simulink model "ASM1_Influentmodel1_ff_calibration"  (Simulink 8.0)
settings: Solver=ode45  StartTime=0.0  StopTime=146  RelTol=1e-5
undefined symbols (not defined in the file or in its folder): Ccj_gperPEperd, Ccj_HH_max, Ccj_HH_min, Ccj_HH_ns, Ccj_HH_nv, Ccj_HH_st, Cli_gperPEperd, Cli_HH_max, Cli_HH_min, Cli_HH_ns, Cli_HH_nv, Cli_HH_st, CODpart_gperPEperd, CODpart_HH_max, CODpart_HH_min, CODpart_HH_ns, CODpart_HH_nv, CODpart_HH_st, CODpart_Ind_kgperd, CODpart_Ind_max, CODpart_Ind_min, CODpart_Ind_ns, CODpart_Ind_nv, CODpart_Ind_st, CODsol_gperPEperd, CODsol_HH_max, CODsol_HH_min, CODsol_HH_ns, CODsol_HH_nv, CODsol_HH_st, CODsol_Ind_kgperd, CODsol_Ind_max, CODsol_Ind_min, CODsol_Ind_ns, CODsol_Ind_nv, CODsol_Ind_st, Csl_gperPEperd, Csl_HH_max, Csl_HH_min, Csl_HH_ns, Csl_HH_nv, Csl_HH_st, Csl_i_gperPEperd, Csl_i_HH_max, Csl_i_HH_min, Csl_i_HH_ns, Csl_i_HH_nv, Csl_i_HH_st, FFfraction, HHpolnoiseswitch, HHpopswitch, Indpolnoiseswitch, Indpopswitch, PE, polnoiseswitch, SI_max, SI_min, SI_ns, SI_nv, SI_st ... (+73)
Description:
  | BSM2 influent model, version 15 March 2005
settings Model: Creator=Krist V. Gernaey  LastModifiedBy=lasn  ExtModeAutoUpdateStatusClock=off
settings DataIOCC: LimitDataPoints=off  SignalLoggingSaveFormat=ModelDataLogs  SignalLoggingName=sigsOut  OutputOption=SpecifiedOutputTimes  OutputTimes=[0:1/96:146]
settings OptimizationCC: InitFltsAndDblsToZero=on
settings DebuggingCC: SaveWithParameterizedLinksMsg=none  SignalResolutionControl=TryResolveAllWithWarning  SolverPrmCheckMsg=none  MultiTaskDSMMsg=warning  MultiTaskCondExecSysMsg=none  FcnCallInpInsideContextMsg=UseLocalSettings  StrictBusMsg=None
settings HardwareCC: TargetEndianess=LittleEndian  TargetHWDeviceType=MATLAB Host  ProdEqTarget=off
settings RTWCC: IncludeERTFirstTime=on
settings GRTTargetCC: CombineOutputUpdateFcns=off  GRTInterface=on

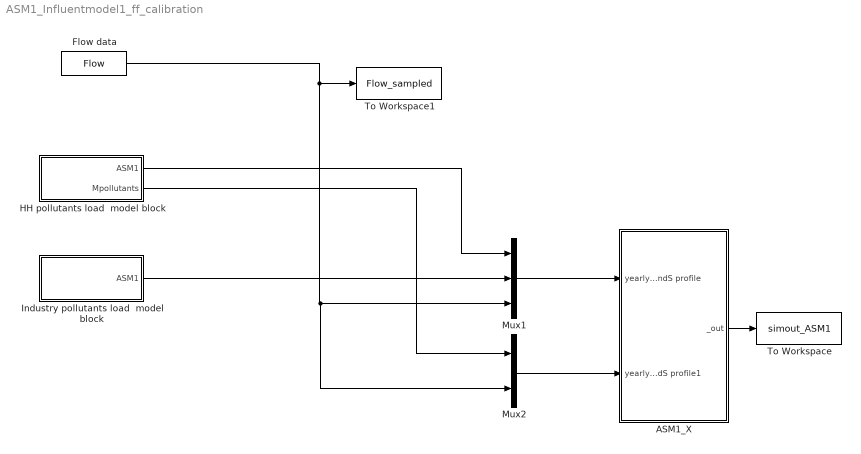
== system ASM1_Influentmodel1_ff_calibration ==
  ASM1_X : Subsystem
  Flow data : FromWorkspace  VariableName=Flow  SampleTime=(1/24)
  "HH pollutants load  model block " : Subsystem
  "Industry pollutants load  model block " : Subsystem
  Mux1 : Mux  Inputs=3
  Mux2 : Mux  Inputs=2
  To Workspace : ToWorkspace  VariableName=simout_ASM1  SampleTime=-1
  To Workspace1 : ToWorkspace  VariableName=Flow_sampled  SampleTime=-1
  wires:
  "HH pollutants load  model block "/1(ASM1) -> Mux1/1
  Mux1/1 -> ASM1_X/1(yearly_indS profile)
  ASM1_X/1(_out) -> To Workspace/1
  "HH pollutants load  model block "/2(Mpollutants) -> Mux2/1
  Mux2/1 -> ASM1_X/2(yearly_indS profile1)
  Flow data/1 -> To Workspace1/1, Mux2/2, Mux1/3
  "Industry pollutants load  model block "/1(ASM1) -> Mux1/2

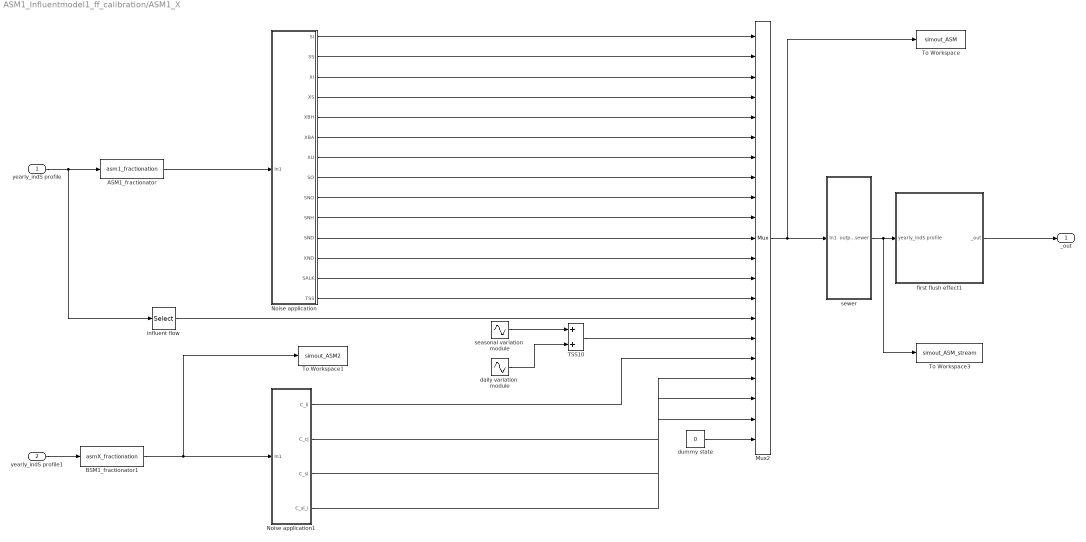
== system ASM1_Influentmodel1_ff_calibration/ASM1_X ==
  yearly_indS profile : Inport
  yearly_indS profile1 : Inport  Port=2
  ASM1_fractionator : S-Function  FunctionName=asm1_fractionation  Parameters=ASM1_PARS, ASM1_FRACTIONS  EnableBusSupport=off
  BSM1_fractionator1 : S-Function  FunctionName=asmX_fractionation  EnableBusSupport=off
  Mux2 : Mux  Inputs=21
  Noise application : Subsystem
  Noise application1 : Subsystem
  TSS10 : Sum
  To Workspace : ToWorkspace  VariableName=simout_ASM  SampleTime=-1
  To Workspace1 : ToWorkspace  VariableName=simout_ASM2  SampleTime=-1
  To Workspace3 : ToWorkspace  VariableName=simout_ASM_stream  SampleTime=-1
  daily variation  module : Sin  Amplitude=TdAmp  Bias=TdBias  Frequency=TdFreq  Phase=TdPhase  SampleTime=0
  "dummy state " : Constant  Value=0
  first flush effect1 : Subsystem
  influent flow : Selector  InputPortWidth=11  IndexOptions=Index vector (dialog)  Indices=[11]  OutputSizes=1
  seasonal variation  module : Sin  Amplitude=TAmp  Bias=TBias  Frequency=TFreq  Phase=TPhase  SampleTime=0
  sewer : Subsystem
  _out : Outport
  wires:
  yearly_indS profile/1 -> influent flow/1, ASM1_fractionator/1
  ASM1_fractionator/1 -> Noise application/1(In1)
  Mux2/1 -> sewer/1(In1), To Workspace/1
  Noise application1/1(C_li) -> Mux2/17
  Noise application/2(SS) -> Mux2/2
  Noise application/1(SI) -> Mux2/1
  Noise application/8(SO) -> Mux2/8
  Noise application/9(SNO) -> Mux2/9
  Noise application/10(SNH) -> Mux2/10
  Noise application/11(SND) -> Mux2/11
  Noise application/12(XND) -> Mux2/12
  seasonal variation  module/1 -> TSS10/1
  daily variation  module/1 -> TSS10/2
  TSS10/1 -> Mux2/16
  yearly_indS profile1/1 -> BSM1_fractionator1/1
  BSM1_fractionator1/1 -> Noise application1/1(In1), To Workspace1/1
  Noise application1/2(C_cj) -> Mux2/18
  Noise application1/3(C_sl) -> Mux2/19
  Noise application1/4(C_sl_i) -> Mux2/20
  "dummy state "/1 -> Mux2/21
  Noise application/3(XI) -> Mux2/3
  Noise application/4(XS) -> Mux2/4
  Noise application/5(XBH) -> Mux2/5
  Noise application/6(XBA) -> Mux2/6
  Noise application/7(XU) -> Mux2/7
  Noise application/13(SALK) -> Mux2/13
  Noise application/14(TSS) -> Mux2/14
  influent flow/1 -> Mux2/15
  sewer/1(output sewer) -> To Workspace3/1, first flush effect1/1(yearly_indS profile)
  first flush effect1/1(_out) -> _out/1

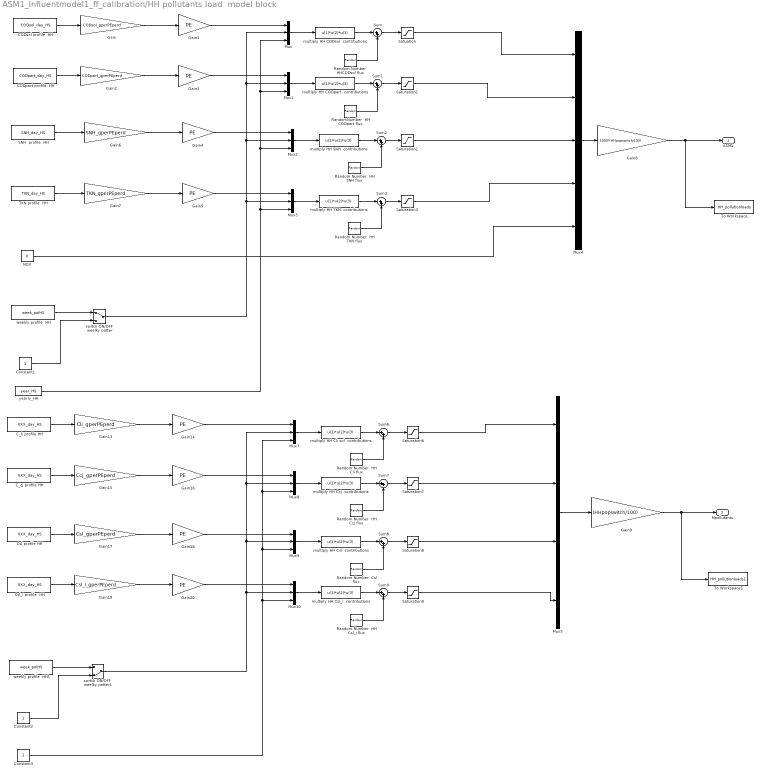
== system ASM1_Influentmodel1_ff_calibration/HH pollutants load  model block  ==
  CODpart profile  HH : FromWorkspace  VariableName=CODpart_day_HS  SampleTime=1/24  Interpolate=off  OutputAfterFinalValue=Cyclic repetition
  CODsol profile  HH : FromWorkspace  VariableName=CODsol_day_HS  SampleTime=1/24  Interpolate=off  OutputAfterFinalValue=Cyclic repetition
  C_cj profile HH : FromWorkspace  VariableName=XXX_day_HS  SampleTime=1/24  Interpolate=off  OutputAfterFinalValue=Cyclic repetition
  C_li profile HH : FromWorkspace  VariableName=XXX_day_HS  SampleTime=1/24  Interpolate=off  OutputAfterFinalValue=Cyclic repetition
  Constant1 : Constant
  Constant2 : Constant
  Constant3 : Constant
  Csl profile HH : FromWorkspace  VariableName=XXX_day_HS  SampleTime=1/24  Interpolate=off  OutputAfterFinalValue=Cyclic repetition
  Csl_I profile  HH : FromWorkspace  VariableName=XXX_day_HS  SampleTime=1/24  Interpolate=off  OutputAfterFinalValue=Cyclic repetition
  Gain : Gain  Gain=CODsol_gperPEperd
  Gain{1,3..5,14,16,18,20} (8 alike) : Gain  Gain=PE
  Gain13 : Gain  Gain=Cli_gperPEperd
  Gain15 : Gain  Gain=Ccj_gperPEperd
  Gain17 : Gain  Gain=Csl_gperPEperd
  Gain19 : Gain  Gain=Csl_i_gperPEperd
  Gain2 : Gain  Gain=CODpart_gperPEperd
  Gain6 : Gain  Gain=SNH_gperPEperd
  Gain7 : Gain  Gain=TKN_gperPEperd
  Gain8 : Gain  Gain=1000*(HHpopswitch/100)
  Gain9 : Gain  Gain=(HHpopswitch/100)
  Mux{,1..3,7..10} (8 alike) : Mux  Inputs=3
  Mux4 : Mux  Inputs=5
  Mux5 : Mux
  NOX : Constant  Value=0
  Random Number  Csl flux : RandomNumber  Variance=Csl_HH_nv*HHpolnoiseswitch  Seed=Csl_HH_ns  SampleTime=Csl_HH_st
  Random Number  HH Ccj flux : RandomNumber  Variance=Ccj_HH_nv*HHpolnoiseswitch  Seed=Ccj_HH_ns  SampleTime=Ccj_HH_st
  Random Number  HH Cli flux : RandomNumber  Variance=Cli_HH_nv*HHpolnoiseswitch  Seed=Cli_HH_ns  SampleTime=Cli_HH_st
  Random Number  HH Csl_i flux : RandomNumber  Variance=Csl_i_HH_nv*HHpolnoiseswitch  Seed=Csl_i_HH_ns  SampleTime=Csl_i_HH_st
  Random Number  HH SNH flux : RandomNumber  Variance=SNH_HH_nv*HHpolnoiseswitch  Seed=SNH_HH_ns  SampleTime=SNH_HH_st
  Random Number  HH TKN flux : RandomNumber  Variance=TKN_HH_nv*HHpolnoiseswitch  Seed=TKN_HH_ns  SampleTime=TKN_HH_st
  Random Number  HHCODsol flux : RandomNumber  Variance=CODsol_HH_nv*HHpolnoiseswitch  Seed=CODsol_HH_ns  SampleTime=CODsol_HH_st
  RandomNumber  HH CODpart flux : RandomNumber  Variance=CODpart_HH_nv*HHpolnoiseswitch  Seed=CODpart_HH_ns  SampleTime=CODpart_HH_st
  SNH  profile  HH : FromWorkspace  VariableName=SNH_day_HS  SampleTime=1/24  Interpolate=off  OutputAfterFinalValue=Cyclic repetition
  Satuation : Saturate  UpperLimit=CODsol_HH_max  LowerLimit=CODsol_HH_min
  Saturation1 : Saturate  UpperLimit=CODpart_HH_max  LowerLimit=CODpart_HH_min
  Saturation2 : Saturate  UpperLimit=SNH_HH_max  LowerLimit=SNH_HH_min
  Saturation3 : Saturate  UpperLimit=TKN_HH_max  LowerLimit=TKN_HH_min
  Saturation6 : Saturate  UpperLimit=Cli_HH_max  LowerLimit=Cli_HH_min
  Saturation7 : Saturate  UpperLimit=Ccj_HH_max  LowerLimit=Ccj_HH_min
  Saturation8 : Saturate  UpperLimit=Csl_HH_max  LowerLimit=Csl_HH_min
  Saturation9 : Saturate  UpperLimit=Csl_i_HH_max  LowerLimit=Csl_i_HH_min
  Sum{,1..3,6..9} (8 alike) : Sum  Inputs=|++
  TKN profile  HH : FromWorkspace  VariableName=TKN_day_HS  SampleTime=1/24  Interpolate=off  OutputAfterFinalValue=Cyclic repetition
  To Workspace : ToWorkspace  VariableName=HH_pollutionloads  SampleTime=-1
  To Workspace1 : ToWorkspace  VariableName=HH_pollutionloads1  SampleTime=-1
  multiply HH CODpart  contributions : Fcn  Expr=u(1)*u(2)*u(3)
  multiply HH CODsol  contributions : Fcn  Expr=u(1)*u(2)*u(3)
  multiply HH Ccj  contributions : Fcn  Expr=u(1)*u(2)*u(3)
  multiply HH Cli sol  contributions : Fcn  Expr=u(1)*u(2)*u(3)
  multiply HH Csl  contributions : Fcn  Expr=u(1)*u(2)*u(3)
  multiply HH Csl_i  contributions : Fcn  Expr=u(1)*u(2)*u(3)
  multiply HH SNH  contributions : Fcn  Expr=u(1)*u(2)*u(3)
  multiply HH TKN  contributions : Fcn  Expr=u(1)*u(2)*u(3)
  switch ON/OFF  weelky patter : ManualSwitch
  switch ON/OFF  weelky patter1 : ManualSwitch  CurrentSetting=0
  weekly profile  HH : FromWorkspace  VariableName=week_polHS  SampleTime=1  Interpolate=off  OutputAfterFinalValue=Cyclic repetition
  weekly profile  HH1 : FromWorkspace  VariableName=week_polHS  SampleTime=1  Interpolate=off  OutputAfterFinalValue=Cyclic repetition
  yearly_HH : FromWorkspace  VariableName=year_HS  SampleTime=1  Interpolate=off  OutputAfterFinalValue=Cyclic repetition
  ASM1 : Outport
  Mpollutants : Outport  Port=2
  wires:
  Random Number  HHCODsol flux/1 -> Sum/2
  CODsol profile  HH/1 -> Gain/1
  Gain/1 -> Gain1/1
  Mux/1 -> multiply HH CODsol  contributions/1
  multiply HH CODsol  contributions/1 -> Sum/1
  Sum/1 -> Satuation/1
  Gain1/1 -> Mux/1
  RandomNumber  HH CODpart flux/1 -> Sum1/2
  CODpart profile  HH/1 -> Gain2/1
  Gain2/1 -> Gain3/1
  Mux1/1 -> multiply HH CODpart  contributions/1
  multiply HH CODpart  contributions/1 -> Sum1/1
  Sum1/1 -> Saturation1/1
  Gain3/1 -> Mux1/1
  Random Number  HH SNH flux/1 -> Sum2/2
  SNH  profile  HH/1 -> Gain6/1
  Gain6/1 -> Gain4/1
  Mux2/1 -> multiply HH SNH  contributions/1
  multiply HH SNH  contributions/1 -> Sum2/1
  Sum2/1 -> Saturation2/1
  Gain4/1 -> Mux2/1
  Random Number  HH TKN flux/1 -> Sum3/2
  TKN profile  HH/1 -> Gain7/1
  Gain7/1 -> Gain5/1
  Mux3/1 -> multiply HH TKN  contributions/1
  multiply HH TKN  contributions/1 -> Sum3/1
  Sum3/1 -> Saturation3/1
  Gain5/1 -> Mux3/1
  Mux4/1 -> Gain8/1
  Constant1/1 -> switch ON/OFF  weelky patter/2
  weekly profile  HH/1 -> switch ON/OFF  weelky patter/1
  Satuation/1 -> Mux4/1
  Saturation1/1 -> Mux4/2
  Saturation2/1 -> Mux4/3
  Saturation3/1 -> Mux4/4
  NOX/1 -> Mux4/5
  switch ON/OFF  weelky patter/1 -> Mux2/2, Mux/2, Mux1/2, Mux3/2
  yearly_HH/1 -> Mux2/3, Mux/3, Mux1/3, Mux3/3
  Gain8/1 -> ASM1/1, To Workspace/1
  Random Number  HH Cli flux/1 -> Sum6/2
  C_li profile HH/1 -> Gain13/1
  Gain13/1 -> Gain14/1
  Mux7/1 -> multiply HH Cli sol  contributions/1
  multiply HH Cli sol  contributions/1 -> Sum6/1
  Sum6/1 -> Saturation6/1
  Gain14/1 -> Mux7/1
  Random Number  HH Ccj flux/1 -> Sum7/2
  C_cj profile HH/1 -> Gain15/1
  Gain15/1 -> Gain16/1
  Mux8/1 -> multiply HH Ccj  contributions/1
  multiply HH Ccj  contributions/1 -> Sum7/1
  Sum7/1 -> Saturation7/1
  Gain16/1 -> Mux8/1
  Constant2/1 -> switch ON/OFF  weelky patter1/2
  weekly profile  HH1/1 -> switch ON/OFF  weelky patter1/1
  Random Number  Csl flux/1 -> Sum8/2
  Csl profile HH/1 -> Gain17/1
  Gain17/1 -> Gain18/1
  Mux9/1 -> multiply HH Csl  contributions/1
  multiply HH Csl  contributions/1 -> Sum8/1
  Sum8/1 -> Saturation8/1
  Gain18/1 -> Mux9/1
  Random Number  HH Csl_i flux/1 -> Sum9/2
  Csl_I profile  HH/1 -> Gain19/1
  Gain19/1 -> Gain20/1
  Mux10/1 -> multiply HH Csl_i  contributions/1
  multiply HH Csl_i  contributions/1 -> Sum9/1
  Sum9/1 -> Saturation9/1
  Gain20/1 -> Mux10/1
  switch ON/OFF  weelky patter1/1 -> Mux7/2, Mux8/2, Mux9/2, Mux10/2
  Saturation9/1 -> Mux5/4
  Saturation8/1 -> Mux5/3
  Saturation7/1 -> Mux5/2
  Saturation6/1 -> Mux5/1
  Mux5/1 -> Gain9/1
  Gain9/1 -> Mpollutants/1, To Workspace1/1
  Constant3/1 -> Mux7/3, Mux8/3, Mux9/3, Mux10/3

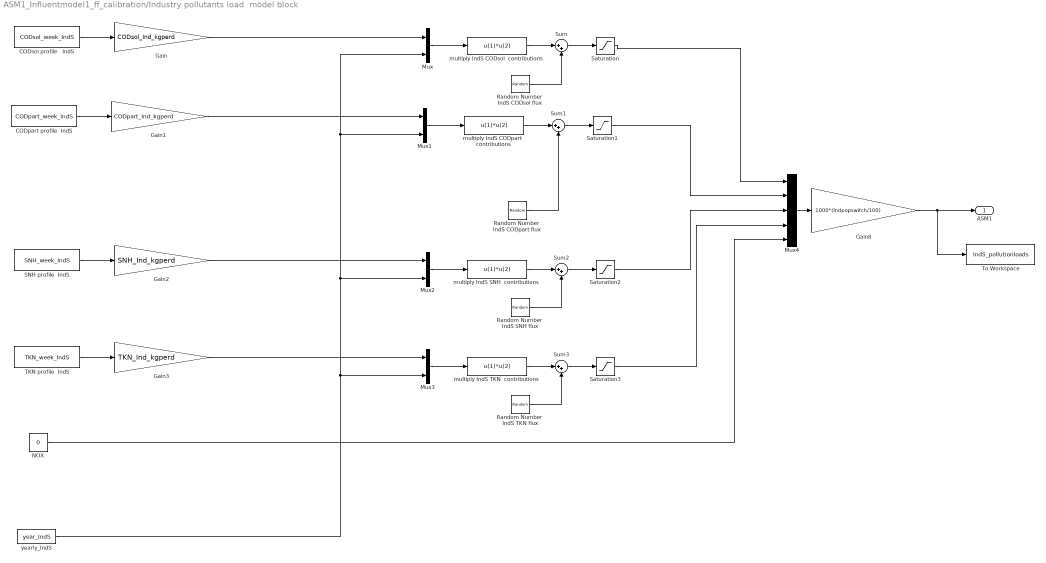
== system ASM1_Influentmodel1_ff_calibration/Industry pollutants load  model block  ==
  CODpart profile  IndS : FromWorkspace  VariableName=CODpart_week_IndS  SampleTime=1/6  Interpolate=off  OutputAfterFinalValue=Cyclic repetition
  CODsol profile   IndS : FromWorkspace  VariableName=CODsol_week_IndS  SampleTime=1/6  Interpolate=off  OutputAfterFinalValue=Cyclic repetition
  Gain : Gain  Gain=CODsol_Ind_kgperd
  Gain1 : Gain  Gain=CODpart_Ind_kgperd
  Gain2 : Gain  Gain=SNH_Ind_kgperd
  Gain3 : Gain  Gain=TKN_Ind_kgperd
  Gain8 : Gain  Gain=1000*(Indpopswitch/100)
  Mux{,1..3} (4 alike) : Mux  Inputs=2
  Mux4 : Mux  Inputs=5
  NOX : Constant  Value=0
  Random Number  IndS CODpart flux : RandomNumber  Variance=CODpart_Ind_nv*Indpolnoiseswitch  Seed=CODpart_Ind_ns  SampleTime=CODpart_Ind_st
  Random Number  IndS CODsol flux : RandomNumber  Variance=CODsol_Ind_nv*Indpolnoiseswitch  Seed=CODsol_Ind_ns  SampleTime=CODsol_Ind_st
  Random Number  IndS SNH flux : RandomNumber  Variance=SNH_Ind_nv*Indpolnoiseswitch  Seed=SNH_Ind_ns  SampleTime=SNH_Ind_st
  Random Number  IndS TKN flux : RandomNumber  Variance=TKN_Ind_nv*Indpolnoiseswitch  Seed=TKN_Ind_ns  SampleTime=TKN_Ind_st
  SNH profile  IndS : FromWorkspace  VariableName=SNH_week_IndS  SampleTime=1/6  Interpolate=off  OutputAfterFinalValue=Cyclic repetition
  Saturation : Saturate  UpperLimit=CODsol_Ind_max  LowerLimit=CODsol_Ind_min
  Saturation1 : Saturate  UpperLimit=CODpart_Ind_max  LowerLimit=CODpart_Ind_min
  Saturation2 : Saturate  UpperLimit=SNH_Ind_max  LowerLimit=SNH_Ind_min
  Saturation3 : Saturate  UpperLimit=TKN_Ind_max  LowerLimit=TKN_Ind_min
  Sum{,1..3} (4 alike) : Sum  Inputs=|++
  TKN profile  IndS : FromWorkspace  VariableName=TKN_week_IndS  SampleTime=1/6  Interpolate=off  OutputAfterFinalValue=Cyclic repetition
  To Workspace : ToWorkspace  VariableName=IndS_pollutionloads  SampleTime=-1
  multiply IndS CODpart  contributions : Fcn  Expr=u(1)*u(2)
  multiply IndS CODsol  contributions : Fcn  Expr=u(1)*u(2)
  multiply IndS SNH  contributions : Fcn  Expr=u(1)*u(2)
  multiply IndS TKN  contributions : Fcn  Expr=u(1)*u(2)
  yearly_IndS : FromWorkspace  VariableName=year_IndS  SampleTime=1  Interpolate=off  OutputAfterFinalValue=Cyclic repetition
  ASM1 : Outport
  wires:
  Random Number  IndS CODsol flux/1 -> Sum/2
  CODsol profile   IndS/1 -> Gain/1
  Mux/1 -> multiply IndS CODsol  contributions/1
  multiply IndS CODsol  contributions/1 -> Sum/1
  Sum/1 -> Saturation/1
  Mux4/1 -> Gain8/1
  Gain/1 -> Mux/1
  Random Number  IndS CODpart flux/1 -> Sum1/2
  CODpart profile  IndS/1 -> Gain1/1
  Mux1/1 -> multiply IndS CODpart  contributions/1
  multiply IndS CODpart  contributions/1 -> Sum1/1
  Sum1/1 -> Saturation1/1
  Gain1/1 -> Mux1/1
  Random Number  IndS SNH flux/1 -> Sum2/2
  SNH profile  IndS/1 -> Gain2/1
  Mux2/1 -> multiply IndS SNH  contributions/1
  multiply IndS SNH  contributions/1 -> Sum2/1
  Sum2/1 -> Saturation2/1
  Gain2/1 -> Mux2/1
  Random Number  IndS TKN flux/1 -> Sum3/2
  TKN profile  IndS/1 -> Gain3/1
  Mux3/1 -> multiply IndS TKN  contributions/1
  multiply IndS TKN  contributions/1 -> Sum3/1
  Sum3/1 -> Saturation3/1
  Gain3/1 -> Mux3/1
  yearly_IndS/1 -> Mux3/2, Mux2/2, Mux/2, Mux1/2
  Saturation/1 -> Mux4/1
  Saturation1/1 -> Mux4/2
  Saturation2/1 -> Mux4/3
  Saturation3/1 -> Mux4/4
  NOX/1 -> Mux4/5
  Gain8/1 -> ASM1/1, To Workspace/1

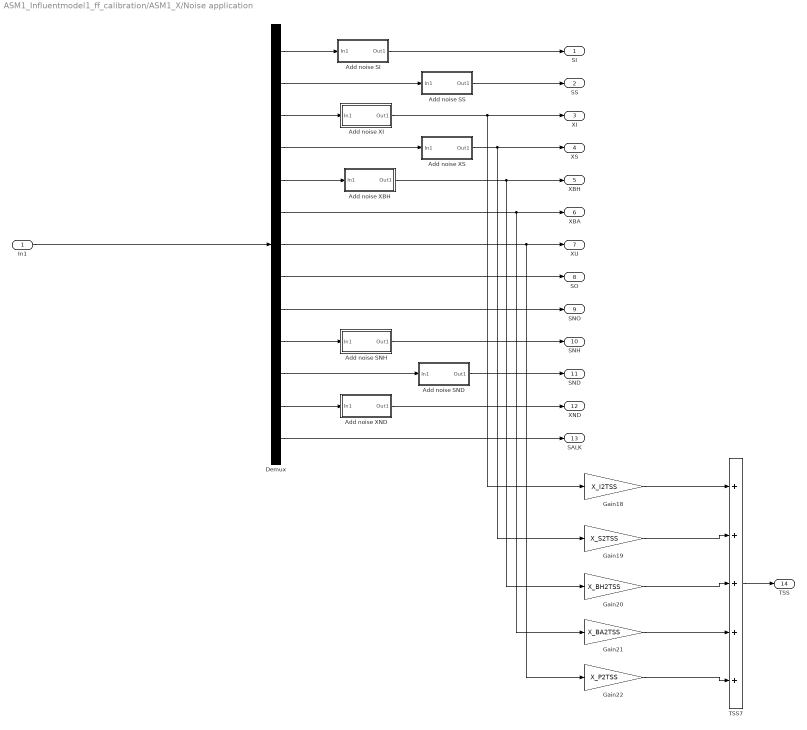
== system ASM1_Influentmodel1_ff_calibration/ASM1_X/Noise application ==
  In1 : Inport
  Add noise SI : Subsystem
  Add noise SND : Subsystem
  Add noise SNH : Subsystem
  Add noise SS : Subsystem
  Add noise XBH : Subsystem
  Add noise XI : Subsystem
  Add noise XND : Subsystem
  Add noise XS : Subsystem
  Demux : Demux  Outputs=[1 1 1 1 1 1 1 1 1 1 1 1 1]
  Gain18 : Gain  Gain=X_I2TSS
  Gain19 : Gain  Gain=X_S2TSS
  Gain20 : Gain  Gain=X_BH2TSS
  Gain21 : Gain  Gain=X_BA2TSS
  Gain22 : Gain  Gain=X_P2TSS
  TSS7 : Sum  Inputs=+++++
  SI : Outport
  SS : Outport  Port=2
  XI : Outport  Port=3
  XS : Outport  Port=4
  XBH : Outport  Port=5
  XBA : Outport  Port=6
  XU : Outport  Port=7
  SO : Outport  Port=8
  SNO : Outport  Port=9
  SNH : Outport  Port=10
  SND : Outport  Port=11
  XND : Outport  Port=12
  SALK : Outport  Port=13
  TSS : Outport  Port=14
  wires:
  In1/1 -> Demux/1
  Demux/1 -> Add noise SI/1(In1)
  Demux/2 -> Add noise SS/1(In1)
  Demux/3 -> Add noise XI/1(In1)
  Demux/4 -> Add noise XS/1(In1)
  Demux/5 -> Add noise XBH/1(In1)
  Demux/6 -> XBA/1, Gain21/1
  Demux/7 -> XU/1, Gain22/1
  Demux/9 -> SNO/1
  Demux/10 -> Add noise SNH/1(In1)
  Demux/11 -> Add noise SND/1(In1)
  Demux/12 -> Add noise XND/1(In1)
  Demux/13 -> SALK/1
  Add noise SI/1(Out1) -> SI/1
  Add noise SS/1(Out1) -> SS/1
  Add noise XI/1(Out1) -> XI/1, Gain18/1
  Add noise XS/1(Out1) -> XS/1, Gain19/1
  Add noise XBH/1(Out1) -> XBH/1, Gain20/1
  Add noise SNH/1(Out1) -> SNH/1
  Add noise SND/1(Out1) -> SND/1
  Add noise XND/1(Out1) -> XND/1
  Demux/8 -> SO/1
  Gain18/1 -> TSS7/1
  Gain20/1 -> TSS7/3
  Gain22/1 -> TSS7/5
  Gain21/1 -> TSS7/4
  Gain19/1 -> TSS7/2
  TSS7/1 -> TSS/1

== system ASM1_Influentmodel1_ff_calibration/ASM1_X/Noise application1 ==
  In1 : Inport
  Demux : Demux  Outputs=[1 1 1 1]
  C_li : Outport
  C_cj : Outport  Port=2
  C_sl : Outport  Port=3
  C_sl_i : Outport  Port=4
  wires:
  In1/1 -> Demux/1
  Demux/1 -> C_li/1
  Demux/2 -> C_cj/1
  Demux/3 -> C_sl/1
  Demux/4 -> C_sl_i/1

== system ASM1_Influentmodel1_ff_calibration/ASM1_X/first flush effect1 ==
  yearly_indS profile : Inport
  Demux : Demux  Outputs=[1 1 1 1 1 1 1 1 1 1 1 1 1 1 1 1 1 1 1 1 1]
  Mux2 : Mux  Inputs=21
  Terminator : Terminator
  first flush effect : Subsystem
  _out : Outport
  wires:
  Demux/1 -> Mux2/1
  Demux/2 -> Mux2/2
  yearly_indS profile/1 -> Demux/1
  Mux2/1 -> _out/1
  Demux/3 -> first flush effect/1(XI_in)
  Demux/4 -> first flush effect/2(XS_in)
  Demux/5 -> first flush effect/3(XBH_in)
  Demux/6 -> first flush effect/4(XBA_in)
  Demux/7 -> first flush effect/5(XU_in)
  Demux/8 -> Mux2/8
  Demux/9 -> Mux2/9
  Demux/10 -> Mux2/10
  Demux/11 -> Mux2/11
  Demux/12 -> first flush effect/6(XND_in)
  Demux/13 -> Mux2/13
  Demux/20 -> first flush effect/8(DX1_in)
  Demux/21 -> first flush effect/9(DX2_in)
  Demux/19 -> Mux2/19
  Demux/18 -> Mux2/18
  Demux/17 -> Mux2/17
  Demux/16 -> Mux2/16
  Demux/15 -> first flush effect/7(Q), Mux2/15
  first flush effect/1(XI_out) -> Mux2/3
  first flush effect/2(XS_out) -> Mux2/4
  first flush effect/3(XBH_out) -> Mux2/5
  first flush effect/4(XBA_out) -> Mux2/6
  first flush effect/5(XU_out) -> Mux2/7
  first flush effect/6(XND_out) -> Mux2/12
  first flush effect/7(XTSS_out) -> Mux2/14
  first flush effect/8(DX1_out) -> Mux2/20
  first flush effect/9(DX2_out) -> Mux2/21
  Demux/14 -> Terminator/1

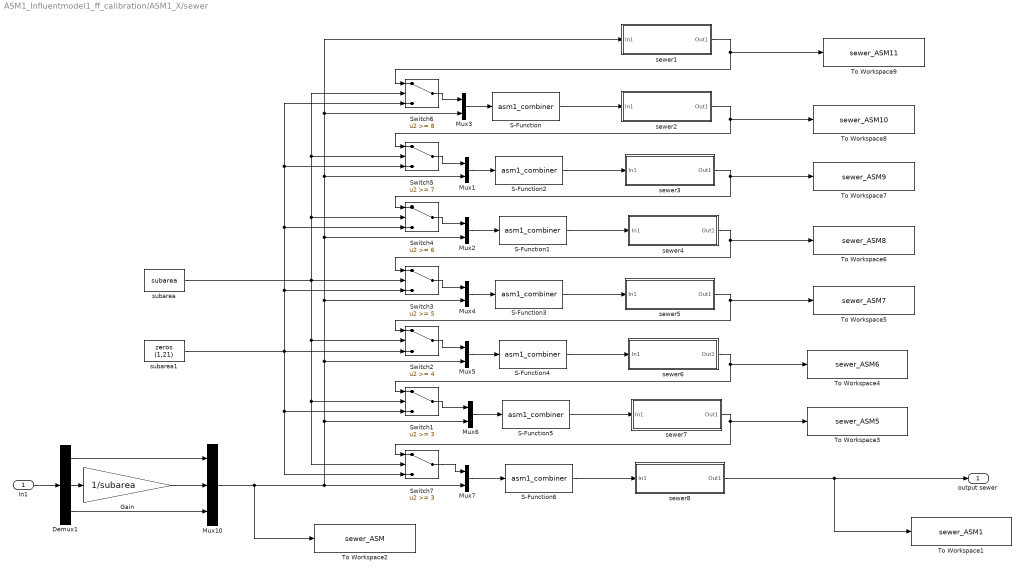
== system ASM1_Influentmodel1_ff_calibration/ASM1_X/sewer ==
  In1 : Inport
  Demux1 : Demux  Outputs=[14 1 6]
  Gain : Gain  Gain=1/subarea
  Mux{1..7} (7 alike) : Mux  Inputs=2
  Mux10 : Mux  Inputs=3
  S-Function{,1..6} (7 alike) : S-Function  FunctionName=asm1_combiner  EnableBusSupport=off
  Switch1 : Switch  Threshold=3  SaturateOnIntegerOverflow=on
  Switch2 : Switch  Threshold=4  SaturateOnIntegerOverflow=on
  Switch3 : Switch  Threshold=5  SaturateOnIntegerOverflow=on
  Switch4 : Switch  Threshold=6  SaturateOnIntegerOverflow=on
  Switch5 : Switch  Threshold=7  SaturateOnIntegerOverflow=on
  Switch6 : Switch  Threshold=8  SaturateOnIntegerOverflow=on
  Switch7 : Switch  Threshold=3  SaturateOnIntegerOverflow=on
  To Workspace1 : ToWorkspace  VariableName=sewer_ASM1  SampleTime=-1
  To Workspace2 : ToWorkspace  VariableName=sewer_ASM  SampleTime=-1
  To Workspace3 : ToWorkspace  VariableName=sewer_ASM5  SampleTime=-1
  To Workspace4 : ToWorkspace  VariableName=sewer_ASM6  SampleTime=-1
  To Workspace5 : ToWorkspace  VariableName=sewer_ASM7  SampleTime=-1
  To Workspace6 : ToWorkspace  VariableName=sewer_ASM8  SampleTime=-1
  To Workspace7 : ToWorkspace  VariableName=sewer_ASM9  SampleTime=-1
  To Workspace8 : ToWorkspace  VariableName=sewer_ASM10  SampleTime=-1
  To Workspace9 : ToWorkspace  VariableName=sewer_ASM11  SampleTime=-1
  sewer1 : Subsystem
  sewer2 : Subsystem
  sewer3 : Subsystem
  sewer4 : Subsystem
  sewer5 : Subsystem
  sewer6 : Subsystem
  sewer7 : Subsystem
  sewer8 : Subsystem
  subarea : Constant  Value=subarea
  subarea1 : Constant  Value=zeros (1,21)
  output sewer : Outport
  wires:
  In1/1 -> Demux1/1
  Demux1/2 -> Gain/1
  Demux1/1 -> Mux10/1
  Demux1/3 -> Mux10/3
  Gain/1 -> Mux10/2
  S-Function/1 -> sewer2/1(In1)
  sewer2/1(Out1) -> Switch5/1, To Workspace8/1
  S-Function2/1 -> sewer3/1(In1)
  sewer3/1(Out1) -> Switch4/1, To Workspace7/1
  S-Function1/1 -> sewer4/1(In1)
  sewer4/1(Out1) -> Switch3/1, To Workspace6/1
  S-Function3/1 -> sewer5/1(In1)
  sewer5/1(Out1) -> Switch2/1, To Workspace5/1
  sewer1/1(Out1) -> Switch6/1, To Workspace9/1
  S-Function4/1 -> sewer6/1(In1)
  sewer6/1(Out1) -> Switch1/1, To Workspace4/1
  S-Function5/1 -> sewer7/1(In1)
  sewer7/1(Out1) -> Switch7/1, To Workspace3/1
  S-Function6/1 -> sewer8/1(In1)
  Mux10/1 -> Mux1/2, Mux3/2, sewer1/1(In1), Mux2/2, Mux4/2, Mux5/2, Mux6/2, Mux7/2, To Workspace2/1
  Switch6/1 -> Mux3/1
  Mux3/1 -> S-Function/1
  Switch5/1 -> Mux1/1
  Switch4/1 -> Mux2/1
  Switch3/1 -> Mux4/1
  Switch1/1 -> Mux6/1
  Switch2/1 -> Mux5/1
  Switch7/1 -> Mux7/1
  Mux1/1 -> S-Function2/1
  Mux2/1 -> S-Function1/1
  Mux4/1 -> S-Function3/1
  Mux5/1 -> S-Function4/1
  Mux6/1 -> S-Function5/1
  Mux7/1 -> S-Function6/1
  sewer8/1(Out1) -> output sewer/1, To Workspace1/1
  subarea/1 -> Switch3/2, Switch6/2, Switch5/2, Switch4/2, Switch2/2, Switch7/2, Switch1/2
  subarea1/1 -> Switch2/3, Switch6/3, Switch5/3, Switch4/3, Switch3/3, Switch1/3, Switch7/3

== system ASM1_Influentmodel1_ff_calibration/ASM1_X/Noise application/Add noise SI ==
  In1 : Inport
  Random Number : RandomNumber  Variance=SI_nv*polnoiseswitch  Seed=SI_ns  SampleTime=SI_st
  Saturation : Saturate  UpperLimit=SI_max  LowerLimit=SI_min
  Sum : Sum  Inputs=|++  SaturateOnIntegerOverflow=on
  Out1 : Outport
  wires:
  Sum/1 -> Saturation/1
  Random Number/1 -> Sum/2
  Saturation/1 -> Out1/1
  In1/1 -> Sum/1

== system ASM1_Influentmodel1_ff_calibration/ASM1_X/Noise application/Add noise SND ==
  In1 : Inport
  Random Number : RandomNumber  Variance=SND_nv*polnoiseswitch  Seed=SND_ns  SampleTime=SND_st
  Saturation : Saturate  UpperLimit=SND_max  LowerLimit=SND_min
  Sum : Sum  Inputs=|++  SaturateOnIntegerOverflow=on
  Out1 : Outport
  wires:
  Sum/1 -> Saturation/1
  Random Number/1 -> Sum/2
  Saturation/1 -> Out1/1
  In1/1 -> Sum/1

== system ASM1_Influentmodel1_ff_calibration/ASM1_X/Noise application/Add noise SNH ==
  In1 : Inport
  Random Number : RandomNumber  Variance=SNH_nv*polnoiseswitch  Seed=SNH_ns  SampleTime=SNH_st
  Saturation : Saturate  UpperLimit=SNH_max  LowerLimit=SNH_min
  Sum : Sum  Inputs=|++  SaturateOnIntegerOverflow=on
  Out1 : Outport
  wires:
  Sum/1 -> Saturation/1
  Random Number/1 -> Sum/2
  Saturation/1 -> Out1/1
  In1/1 -> Sum/1

== system ASM1_Influentmodel1_ff_calibration/ASM1_X/Noise application/Add noise SS ==
  In1 : Inport
  Random Number : RandomNumber  Variance=SS_nv*polnoiseswitch  Seed=SS_ns  SampleTime=SS_st
  Saturation : Saturate  UpperLimit=SS_max  LowerLimit=SS_min
  Sum : Sum  Inputs=|++  SaturateOnIntegerOverflow=on
  Out1 : Outport
  wires:
  Sum/1 -> Saturation/1
  Random Number/1 -> Sum/2
  Saturation/1 -> Out1/1
  In1/1 -> Sum/1

== system ASM1_Influentmodel1_ff_calibration/ASM1_X/Noise application/Add noise XBH ==
  In1 : Inport
  Random Number : RandomNumber  Variance=XBH_nv*polnoiseswitch  Seed=XBH_ns  SampleTime=XBH_st
  Saturation : Saturate  UpperLimit=XBH_max  LowerLimit=XBH_min
  Sum : Sum  Inputs=|++  SaturateOnIntegerOverflow=on
  Out1 : Outport
  wires:
  Sum/1 -> Saturation/1
  Random Number/1 -> Sum/2
  Saturation/1 -> Out1/1
  In1/1 -> Sum/1

== system ASM1_Influentmodel1_ff_calibration/ASM1_X/Noise application/Add noise XI ==
  In1 : Inport
  Random Number : RandomNumber  Variance=XI_nv*polnoiseswitch  Seed=XI_ns  SampleTime=XI_st
  Saturation : Saturate  UpperLimit=XI_max  LowerLimit=XI_min
  Sum : Sum  Inputs=|++  SaturateOnIntegerOverflow=on
  Out1 : Outport
  wires:
  Sum/1 -> Saturation/1
  Random Number/1 -> Sum/2
  Saturation/1 -> Out1/1
  In1/1 -> Sum/1

== system ASM1_Influentmodel1_ff_calibration/ASM1_X/Noise application/Add noise XND ==
  In1 : Inport
  Random Number : RandomNumber  Variance=XND_nv*polnoiseswitch  Seed=XND_ns  SampleTime=XND_st
  Saturation : Saturate  UpperLimit=XND_max  LowerLimit=XND_min
  Sum : Sum  Inputs=|++  SaturateOnIntegerOverflow=on
  Out1 : Outport
  wires:
  Sum/1 -> Saturation/1
  Random Number/1 -> Sum/2
  Saturation/1 -> Out1/1
  In1/1 -> Sum/1

== system ASM1_Influentmodel1_ff_calibration/ASM1_X/Noise application/Add noise XS ==
  In1 : Inport
  Random Number : RandomNumber  Variance=XS_nv*polnoiseswitch  Seed=XS_ns  SampleTime=XS_st
  Saturation : Saturate  UpperLimit=XS_max  LowerLimit=XS_min
  Sum : Sum  Inputs=|++  SaturateOnIntegerOverflow=on
  Out1 : Outport
  wires:
  Sum/1 -> Saturation/1
  Random Number/1 -> Sum/2
  Saturation/1 -> Out1/1
  In1/1 -> Sum/1

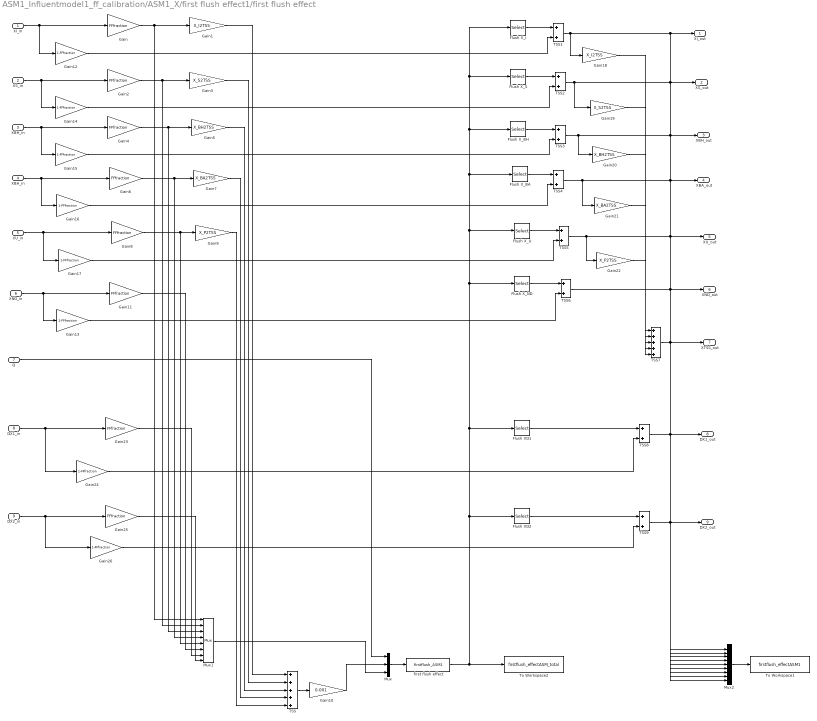
== system ASM1_Influentmodel1_ff_calibration/ASM1_X/first flush effect1/first flush effect ==
  XI_in : Inport
  XS_in : Inport  Port=2
  XBH_in : Inport  Port=3
  XBA_in : Inport  Port=4
  XU_in : Inport  Port=5
  XND_in : Inport  Port=6
  Q : Inport  Port=7
  DX1_in : Inport  Port=8
  DX2_in : Inport  Port=9
  Flush XD1 : Selector  InputPortWidth=19  IndexOptions=Index vector (dialog)  Indices=[9]  OutputSizes=1
  Flush XD2 : Selector  InputPortWidth=19  IndexOptions=Index vector (dialog)  Indices=[10]  OutputSizes=1
  Flush X_BA : Selector  InputPortWidth=19  IndexOptions=Index vector (dialog)  Indices=[6]  OutputSizes=1
  Flush X_BH : Selector  InputPortWidth=19  IndexOptions=Index vector (dialog)  Indices=[5]  OutputSizes=1
  Flush X_I : Selector  InputPortWidth=19  IndexOptions=Index vector (dialog)  Indices=[3]  OutputSizes=1
  Flush X_ND : Selector  InputPortWidth=19  IndexOptions=Index vector (dialog)  Indices=[8]  OutputSizes=1
  Flush X_S : Selector  InputPortWidth=19  IndexOptions=Index vector (dialog)  Indices=[4]  OutputSizes=1
  Flush X_U : Selector  InputPortWidth=19  IndexOptions=Index vector (dialog)  Indices=[7]  OutputSizes=1
  Gain{,2,4,6,8,11,23,25} (8 alike) : Gain  Gain=FFfraction
  Gain1 : Gain  Gain=X_I2TSS
  Gain10 : Gain  Gain=0.001
  Gain{12..17,24,26} (8 alike) : Gain  Gain=1-FFfraction
  Gain18 : Gain  Gain=X_I2TSS
  Gain19 : Gain  Gain=X_S2TSS
  Gain20 : Gain  Gain=X_BH2TSS
  Gain21 : Gain  Gain=X_BA2TSS
  Gain22 : Gain  Gain=X_P2TSS
  Gain3 : Gain  Gain=X_S2TSS
  Gain5 : Gain  Gain=X_BH2TSS
  Gain7 : Gain  Gain=X_BA2TSS
  Gain9 : Gain  Gain=X_P2TSS
  Mux : Mux  Inputs=3
  Mux1 : Mux  Inputs=8
  Mux2 : Mux  Inputs=9
  TSS : Sum  Inputs=+++++
  TSS{1..6,8..9} (8 alike) : Sum
  TSS7 : Sum  Inputs=+++++
  To Workspace1 : ToWorkspace  VariableName=firstflush_effectASM1  SampleTime=-1
  To Workspace2 : ToWorkspace  VariableName=firstflush_effectASM_total  SampleTime=-1
  first flush effect : S-Function  FunctionName=firstflush_ASM1  Parameters=ASM1_XINIT, SSPARS  EnableBusSupport=off
  XI_out : Outport
  XS_out : Outport  Port=2
  XBH_out : Outport  Port=3
  XBA_out : Outport  Port=4
  XU_out : Outport  Port=5
  XND_out : Outport  Port=6
  XTSS_out : Outport  Port=7
  DX1_out : Outport  Port=8
  DX2_out : Outport  Port=9
  wires:
  XI_in/1 -> Gain/1, Gain12/1
  Gain/1 -> Gain1/1, Mux1/1
  XS_in/1 -> Gain2/1, Gain14/1
  Gain2/1 -> Gain3/1, Mux1/2
  XBH_in/1 -> Gain4/1, Gain15/1
  Gain4/1 -> Gain5/1, Mux1/3
  XBA_in/1 -> Gain6/1, Gain16/1
  Gain6/1 -> Gain7/1, Mux1/4
  XU_in/1 -> Gain8/1, Gain17/1
  Gain8/1 -> Gain9/1, Mux1/5
  Gain11/1 -> Mux1/6
  XND_in/1 -> Gain11/1, Gain13/1
  Gain12/1 -> TSS1/2
  Flush X_I/1 -> TSS1/1
  Flush X_S/1 -> TSS2/1
  Gain14/1 -> TSS2/2
  Flush X_BH/1 -> TSS3/1
  Gain15/1 -> TSS3/2
  Gain16/1 -> TSS4/2
  Flush X_BA/1 -> TSS4/1
  Gain17/1 -> TSS5/2
  Flush X_U/1 -> TSS5/1
  Gain13/1 -> TSS6/2
  Flush X_ND/1 -> TSS6/1
  TSS1/1 -> Gain18/1, XI_out/1, Mux2/1
  TSS2/1 -> Gain19/1, XS_out/1, Mux2/2
  TSS3/1 -> Gain20/1, XBH_out/1, Mux2/3
  TSS4/1 -> Gain21/1, XBA_out/1, Mux2/4
  TSS5/1 -> Gain22/1, XU_out/1, Mux2/5
  TSS6/1 -> XND_out/1, Mux2/6
  Gain18/1 -> TSS7/1
  Gain19/1 -> TSS7/2
  Gain20/1 -> TSS7/3
  Gain21/1 -> TSS7/4
  Gain22/1 -> TSS7/5
  TSS7/1 -> XTSS_out/1, Mux2/7
  Mux2/1 -> To Workspace1/1
  DX1_in/1 -> Gain23/1, Gain24/1
  DX2_in/1 -> Gain25/1, Gain26/1
  Gain1/1 -> TSS/1
  Gain3/1 -> TSS/2
  Gain5/1 -> TSS/3
  Gain7/1 -> TSS/4
  Gain9/1 -> TSS/5
  Mux1/1 -> Mux/3
  Q/1 -> Mux/1
  Mux/1 -> first flush effect/1
  TSS/1 -> Gain10/1
  Gain10/1 -> Mux/2
  first flush effect/1 -> Flush X_I/1, Flush X_S/1, Flush X_BH/1, Flush X_BA/1, Flush X_U/1, Flush X_ND/1, Flush XD1/1, Flush XD2/1, To Workspace2/1
  Gain24/1 -> TSS8/2
  TSS8/1 -> DX1_out/1, Mux2/8
  Gain26/1 -> TSS9/2
  TSS9/1 -> DX2_out/1, Mux2/9
  Gain23/1 -> Mux1/7
  Gain25/1 -> Mux1/8
  Flush XD2/1 -> TSS9/1
  Flush XD1/1 -> TSS8/1

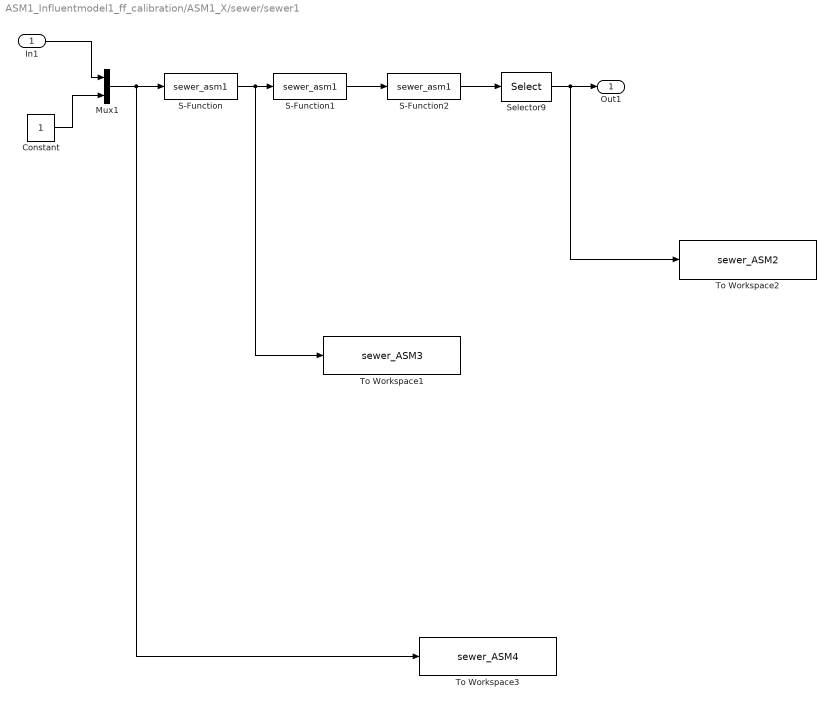
== system ASM1_Influentmodel1_ff_calibration/ASM1_X/sewer/sewer1 ==
  In1 : Inport
  Constant : Constant
  Mux1 : Mux  Inputs=2
  S-Function : S-Function  FunctionName=sewer_asm1  Parameters=ASM1_SEWERINIT, ASM1_PARS, SPAR, SOSAT, ASMX, KLa  EnableBusSupport=off
  S-Function1 : S-Function  FunctionName=sewer_asm1  Parameters=ASM1_SEWERINIT, ASM1_PARS, SPAR, SOSAT, ASMX, KLa  EnableBusSupport=off
  S-Function2 : S-Function  FunctionName=sewer_asm1  Parameters=ASM1_SEWERINIT, ASM1_PARS, SPAR, SOSAT, ASMX, KLa  EnableBusSupport=off
  Selector9 : Selector  InputPortWidth=22  IndexOptions=Index vector (dialog)  Indices=[1 2 3 4 5 6 7 8 9 10 11 12 13 14 15 16 17 18 19 20 21]  OutputSizes=1
  To Workspace1 : ToWorkspace  VariableName=sewer_ASM3  SampleTime=-1
  To Workspace2 : ToWorkspace  VariableName=sewer_ASM2  SampleTime=-1
  To Workspace3 : ToWorkspace  VariableName=sewer_ASM4  SampleTime=-1
  Out1 : Outport
  wires:
  S-Function/1 -> S-Function1/1, To Workspace1/1
  S-Function1/1 -> S-Function2/1
  S-Function2/1 -> Selector9/1
  Mux1/1 -> S-Function/1, To Workspace3/1
  Constant/1 -> Mux1/2
  In1/1 -> Mux1/1
  Selector9/1 -> Out1/1, To Workspace2/1

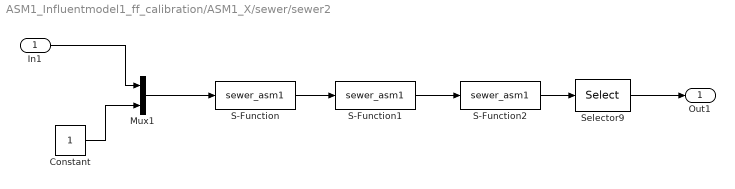
== system ASM1_Influentmodel1_ff_calibration/ASM1_X/sewer/sewer2 ==
  In1 : Inport
  Constant : Constant
  Mux1 : Mux  Inputs=2
  S-Function : S-Function  FunctionName=sewer_asm1  Parameters=ASM1_SEWERINIT, ASM1_PARS, SPAR, SOSAT, ASMX, KLa  EnableBusSupport=off
  S-Function1 : S-Function  FunctionName=sewer_asm1  Parameters=ASM1_SEWERINIT, ASM1_PARS, SPAR, SOSAT, ASMX, KLa  EnableBusSupport=off
  S-Function2 : S-Function  FunctionName=sewer_asm1  Parameters=ASM1_SEWERINIT, ASM1_PARS, SPAR, SOSAT, ASMX, KLa  EnableBusSupport=off
  Selector9 : Selector  InputPortWidth=22  IndexOptions=Index vector (dialog)  Indices=[1 2 3 4 5 6 7 8 9 10 11 12 13 14 15 16 17 18 19 20 21]  OutputSizes=1
  Out1 : Outport
  wires:
  Constant/1 -> Mux1/2
  Selector9/1 -> Out1/1
  In1/1 -> Mux1/1
  S-Function/1 -> S-Function1/1
  S-Function1/1 -> S-Function2/1
  Mux1/1 -> S-Function/1
  S-Function2/1 -> Selector9/1

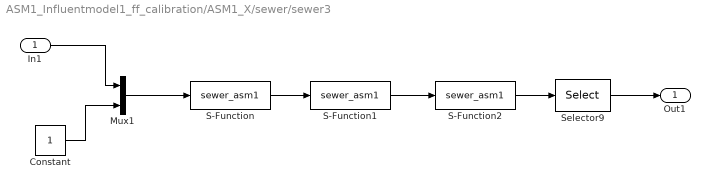
== system ASM1_Influentmodel1_ff_calibration/ASM1_X/sewer/sewer3 ==
  In1 : Inport
  Constant : Constant
  Mux1 : Mux  Inputs=2
  S-Function : S-Function  FunctionName=sewer_asm1  Parameters=ASM1_SEWERINIT, ASM1_PARS, SPAR, SOSAT, ASMX, KLa  EnableBusSupport=off
  S-Function1 : S-Function  FunctionName=sewer_asm1  Parameters=ASM1_SEWERINIT, ASM1_PARS, SPAR, SOSAT, ASMX, KLa  EnableBusSupport=off
  S-Function2 : S-Function  FunctionName=sewer_asm1  Parameters=ASM1_SEWERINIT, ASM1_PARS, SPAR, SOSAT, ASMX, KLa  EnableBusSupport=off
  Selector9 : Selector  InputPortWidth=22  IndexOptions=Index vector (dialog)  Indices=[1 2 3 4 5 6 7 8 9 10 11 12 13 14 15 16 17 18 19 20 21]  OutputSizes=1
  Out1 : Outport
  wires:
  Constant/1 -> Mux1/2
  In1/1 -> Mux1/1
  Selector9/1 -> Out1/1
  S-Function/1 -> S-Function1/1
  S-Function1/1 -> S-Function2/1
  S-Function2/1 -> Selector9/1
  Mux1/1 -> S-Function/1

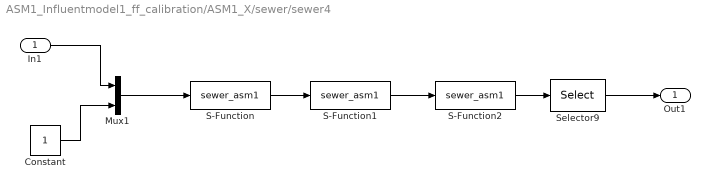
== system ASM1_Influentmodel1_ff_calibration/ASM1_X/sewer/sewer4 ==
  In1 : Inport
  Constant : Constant
  Mux1 : Mux  Inputs=2
  S-Function : S-Function  FunctionName=sewer_asm1  Parameters=ASM1_SEWERINIT, ASM1_PARS, SPAR, SOSAT, ASMX, KLa  EnableBusSupport=off
  S-Function1 : S-Function  FunctionName=sewer_asm1  Parameters=ASM1_SEWERINIT, ASM1_PARS, SPAR, SOSAT, ASMX, KLa  EnableBusSupport=off
  S-Function2 : S-Function  FunctionName=sewer_asm1  Parameters=ASM1_SEWERINIT, ASM1_PARS, SPAR, SOSAT, ASMX, KLa  EnableBusSupport=off
  Selector9 : Selector  InputPortWidth=22  IndexOptions=Index vector (dialog)  Indices=[1 2 3 4 5 6 7 8 9 10 11 12 13 14 15 16 17 18 19 20 21]  OutputSizes=1
  Out1 : Outport
  wires:
  Constant/1 -> Mux1/2
  In1/1 -> Mux1/1
  Selector9/1 -> Out1/1
  S-Function/1 -> S-Function1/1
  S-Function1/1 -> S-Function2/1
  S-Function2/1 -> Selector9/1
  Mux1/1 -> S-Function/1

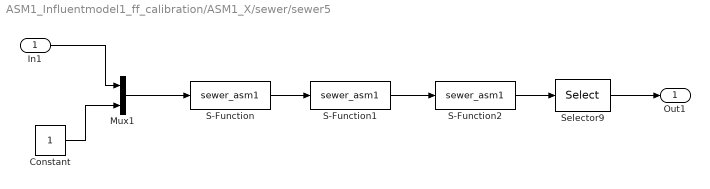
== system ASM1_Influentmodel1_ff_calibration/ASM1_X/sewer/sewer5 ==
  In1 : Inport
  Constant : Constant
  Mux1 : Mux  Inputs=2
  S-Function : S-Function  FunctionName=sewer_asm1  Parameters=ASM1_SEWERINIT, ASM1_PARS, SPAR, SOSAT, ASMX, KLa  EnableBusSupport=off
  S-Function1 : S-Function  FunctionName=sewer_asm1  Parameters=ASM1_SEWERINIT, ASM1_PARS, SPAR, SOSAT, ASMX, KLa  EnableBusSupport=off
  S-Function2 : S-Function  FunctionName=sewer_asm1  Parameters=ASM1_SEWERINIT, ASM1_PARS, SPAR, SOSAT, ASMX, KLa  EnableBusSupport=off
  Selector9 : Selector  InputPortWidth=22  IndexOptions=Index vector (dialog)  Indices=[1 2 3 4 5 6 7 8 9 10 11 12 13 14 15 16 17 18 19 20 21]  OutputSizes=1
  Out1 : Outport
  wires:
  Constant/1 -> Mux1/2
  In1/1 -> Mux1/1
  Selector9/1 -> Out1/1
  S-Function/1 -> S-Function1/1
  S-Function1/1 -> S-Function2/1
  S-Function2/1 -> Selector9/1
  Mux1/1 -> S-Function/1

== system ASM1_Influentmodel1_ff_calibration/ASM1_X/sewer/sewer6 ==
  In1 : Inport
  Constant : Constant
  Mux1 : Mux  Inputs=2
  S-Function : S-Function  FunctionName=sewer_asm1  Parameters=ASM1_SEWERINIT, ASM1_PARS, SPAR, SOSAT, ASMX, KLa  EnableBusSupport=off
  S-Function1 : S-Function  FunctionName=sewer_asm1  Parameters=ASM1_SEWERINIT, ASM1_PARS, SPAR, SOSAT, ASMX, KLa  EnableBusSupport=off
  S-Function2 : S-Function  FunctionName=sewer_asm1  Parameters=ASM1_SEWERINIT, ASM1_PARS, SPAR, SOSAT, ASMX, KLa  EnableBusSupport=off
  Selector9 : Selector  InputPortWidth=22  IndexOptions=Index vector (dialog)  Indices=[1 2 3 4 5 6 7 8 9 10 11 12 13 14 15 16 17 18 19 20 21]  OutputSizes=1
  Out1 : Outport
  wires:
  Constant/1 -> Mux1/2
  In1/1 -> Mux1/1
  Selector9/1 -> Out1/1
  S-Function/1 -> S-Function1/1
  S-Function1/1 -> S-Function2/1
  S-Function2/1 -> Selector9/1
  Mux1/1 -> S-Function/1

== system ASM1_Influentmodel1_ff_calibration/ASM1_X/sewer/sewer7 ==
  In1 : Inport
  Constant : Constant
  Mux1 : Mux  Inputs=2
  S-Function : S-Function  FunctionName=sewer_asm1  Parameters=ASM1_SEWERINIT, ASM1_PARS, SPAR, SOSAT, ASMX, KLa  EnableBusSupport=off
  S-Function1 : S-Function  FunctionName=sewer_asm1  Parameters=ASM1_SEWERINIT, ASM1_PARS, SPAR, SOSAT, ASMX, KLa  EnableBusSupport=off
  S-Function2 : S-Function  FunctionName=sewer_asm1  Parameters=ASM1_SEWERINIT, ASM1_PARS, SPAR, SOSAT, ASMX, KLa  EnableBusSupport=off
  Selector9 : Selector  InputPortWidth=22  IndexOptions=Index vector (dialog)  Indices=[1 2 3 4 5 6 7 8 9 10 11 12 13 14 15 16 17 18 19 20 21]  OutputSizes=1
  Out1 : Outport
  wires:
  Constant/1 -> Mux1/2
  In1/1 -> Mux1/1
  Selector9/1 -> Out1/1
  S-Function/1 -> S-Function1/1
  S-Function1/1 -> S-Function2/1
  S-Function2/1 -> Selector9/1
  Mux1/1 -> S-Function/1

== system ASM1_Influentmodel1_ff_calibration/ASM1_X/sewer/sewer8 ==
  In1 : Inport
  Constant : Constant
  Mux1 : Mux  Inputs=2
  S-Function : S-Function  FunctionName=sewer_asm1  Parameters=ASM1_SEWERINIT, ASM1_PARS, SPAR, SOSAT, ASMX, KLa  EnableBusSupport=off
  S-Function1 : S-Function  FunctionName=sewer_asm1  Parameters=ASM1_SEWERINIT, ASM1_PARS, SPAR, SOSAT, ASMX, KLa  EnableBusSupport=off
  S-Function2 : S-Function  FunctionName=sewer_asm1  Parameters=ASM1_SEWERINIT, ASM1_PARS, SPAR, SOSAT, ASMX, KLa  EnableBusSupport=off
  Selector9 : Selector  InputPortWidth=22  IndexOptions=Index vector (dialog)  Indices=[1 2 3 4 5 6 7 8 9 10 11 12 13 14 15 16 17 18 19 20 21 ]  OutputSizes=1
  Out1 : Outport
  wires:
  Constant/1 -> Mux1/2
  In1/1 -> Mux1/1
  Selector9/1 -> Out1/1
  S-Function/1 -> S-Function1/1
  S-Function1/1 -> S-Function2/1
  S-Function2/1 -> Selector9/1
  Mux1/1 -> S-Function/1
